simulink model "PitchRateLimiter_Harness"  (R2023b)
settings: Solver=FixedStepDiscrete  StartTime=0.0  StopTime=2  FixedStep=Sample_time  RelTol=1e-3
model workspace (MAT data in the model file):
  input_valid_test = timeseries
  input_valid_test.Name = 'input_valid_test'
  input_valid_test.DataInfo = tsdata.datametadata
  input_valid_test.DataInfo.Interpolation = tsdata.interpolation
  input_valid_test.DataInfo.Interpolation.Fhandle : function handle (value not decoded)
  input_valid_test.DataInfo.Interpolation.Name = 'linear'
  input_valid_test.TimeInfo = tsdata.timemetadata
  input_valid_test.TimeInfo.Length = 2
  input_valid_test.TimeInfo.DuplicateTimes = 0
  input_valid_test.TimeInfo.Time_ = [0; 0.02]
  input_valid_test.TimeInfo.Initialized = 1
  input_valid_test.QualityInfo = tsdata.qualmetadata
  input_valid_test.Data_ = [1; 1]
  normal_mode_test = timeseries
  normal_mode_test.Name = 'normal_mode_test'
  normal_mode_test.DataInfo = tsdata.datametadata
  normal_mode_test.DataInfo.Interpolation = tsdata.interpolation
  normal_mode_test.DataInfo.Interpolation.Fhandle : function handle (value not decoded)
  normal_mode_test.DataInfo.Interpolation.Name = 'linear'
  normal_mode_test.TimeInfo = tsdata.timemetadata
  normal_mode_test.TimeInfo.Length = 2
  normal_mode_test.TimeInfo.DuplicateTimes = 0
  normal_mode_test.TimeInfo.Time_ = [0; 0.02]
  normal_mode_test.TimeInfo.Initialized = 1
  normal_mode_test.QualityInfo = tsdata.qualmetadata
  normal_mode_test.Data_ = [1; 1]
  q_cmd_test = timeseries
  q_cmd_test.Name = 'q_cmd_test'
  q_cmd_test.DataInfo = tsdata.datametadata
  q_cmd_test.DataInfo.Interpolation = tsdata.interpolation
  q_cmd_test.DataInfo.Interpolation.Fhandle : function handle (value not decoded)
  q_cmd_test.DataInfo.Interpolation.Name = 'linear'
  q_cmd_test.TimeInfo = tsdata.timemetadata
  q_cmd_test.TimeInfo.Length = 2
  q_cmd_test.TimeInfo.DuplicateTimes = 0
  q_cmd_test.TimeInfo.Time_ = [0; 0.02]
  q_cmd_test.TimeInfo.Initialized = 1
  q_cmd_test.QualityInfo = tsdata.qualmetadata
  q_cmd_test.Data_ = [0; 0]
undefined symbols (not defined in the file): Sample_time
Description:
  | Standalone executable harness for PitchRateLimiter. It is used when Simulink Test is unavailable and remains useful for scripted tests.
settings Model: DataDictionary=FCS_Data.sldd  Creator=Tyler  LastModifiedBy=Tyler
settings CodeAppCC: MaxIdLength=63

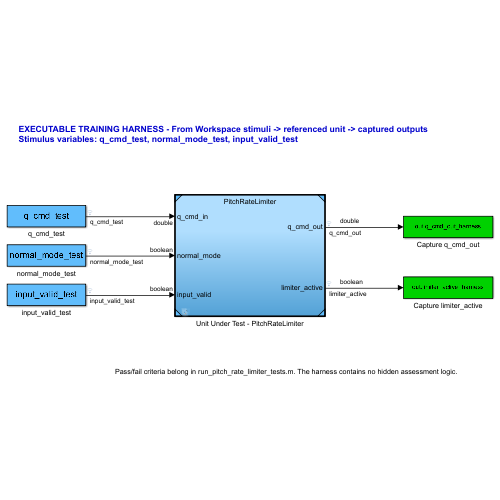
[thumbnail: Simulink's stored preview of the top-level diagram]
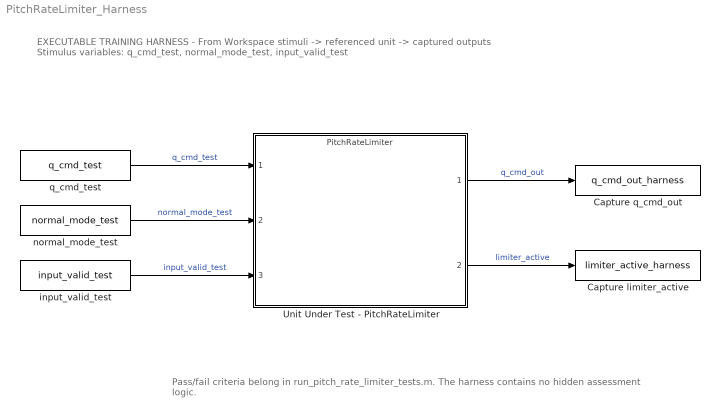
== system PitchRateLimiter_Harness ==
  note: EXECUTABLE TRAINING HARNESS - From Workspace stimuli -> referenced unit -> captured outputs
      | Stimulus variables: q_cmd_test, normal_mode_test, input_valid_test
  note: Pass/fail criteria belong in run_pitch_rate_limiter_tests.m. The harness contains no hidden assessment logic.
  Capture limiter_active : ToWorkspace  VariableName=limiter_active_harness  SaveFormat=Timeseries  SampleTime=-1
  Capture q_cmd_out : ToWorkspace  VariableName=q_cmd_out_harness  SaveFormat=Timeseries  SampleTime=-1
  Unit Under Test - PitchRateLimiter : ModelReference  Description=Model reference to PitchRateLimiter.slx (illustrative training component).  ModelNameDialog=PitchRateLimiter  SimulationMode=Accelerator  ModelReferenceVersion=1.2
  input_valid_test : FromWorkspace  VariableName=input_valid_test  SampleTime=Sample_time  Interpolate=off  OutputAfterFinalValue=Holding final value
  normal_mode_test : FromWorkspace  VariableName=normal_mode_test  SampleTime=Sample_time  Interpolate=off  OutputAfterFinalValue=Holding final value
  q_cmd_test : FromWorkspace  VariableName=q_cmd_test  SampleTime=Sample_time  Interpolate=off  OutputAfterFinalValue=Holding final value
  wires:
  q_cmd_test/1 -> Unit Under Test - PitchRateLimiter/1  "q_cmd_test"
  normal_mode_test/1 -> Unit Under Test - PitchRateLimiter/2  "normal_mode_test"
  input_valid_test/1 -> Unit Under Test - PitchRateLimiter/3  "input_valid_test"
  Unit Under Test - PitchRateLimiter/1 -> Capture q_cmd_out/1  "q_cmd_out"
  Unit Under Test - PitchRateLimiter/2 -> Capture limiter_active/1  "limiter_active"
